simulink model "sim_ismc"  (R2023b)
settings: Solver=ode1  StartTime=0.0  StopTime=2  FixedStep=0.0001  RelTol=1e-3
values from neighbouring files (symbols this model uses):
  dn_lim = -up_lim    (= -10)    [ai_smc.m]    (also in ismc.m; st_smc.m)
  k_smc_e = 1    [ismc.m]
  k_smc_ie = -5    [ismc.m]
  M = -2    [fsmc.m]    (also in ismc.m = 10)
  Te = 0.001    [ai_smc.m]    (also in fsmc.m; ismc.m; st_smc.m)
  Tm = 0.2    [ai_smc.m]    (also in fsmc.m; ismc.m; st_smc.m)
  up_lim = 10    [ai_smc.m]    (also in ismc.m; st_smc.m)
settings Model: Creator=HP  LastModifiedBy=HP

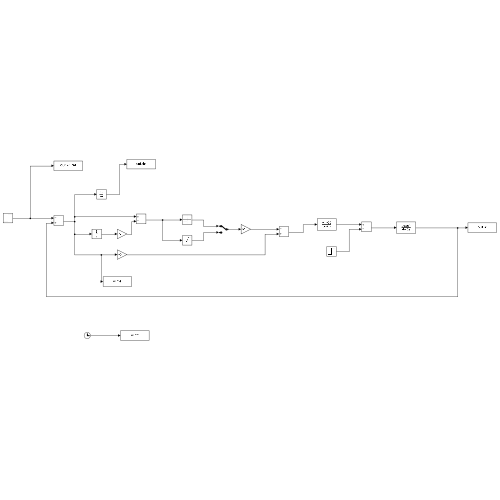
[thumbnail: Simulink's stored preview of the top-level diagram]
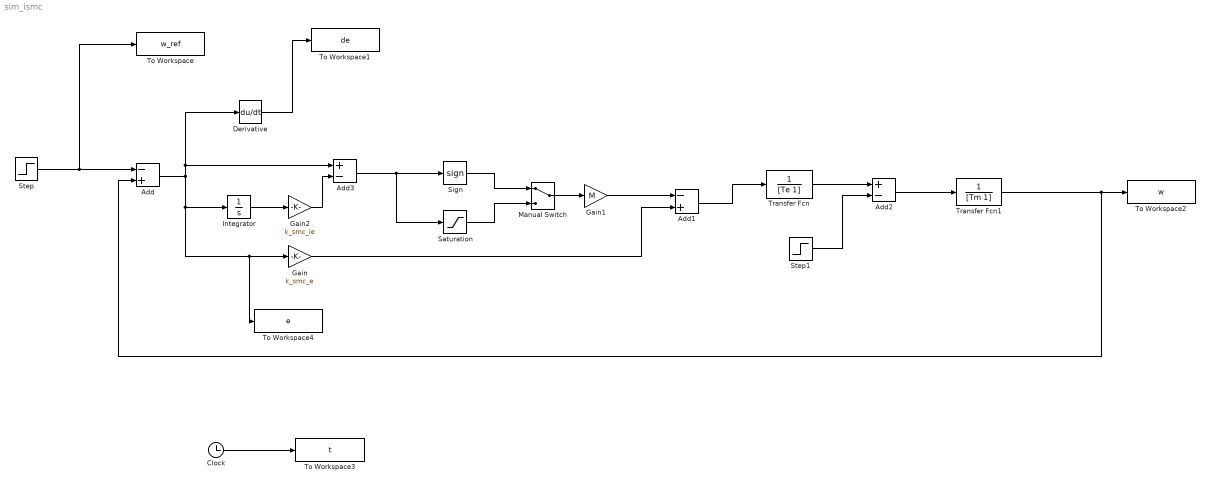
== system sim_ismc ==
  Add : Sum  Inputs=-+
  Add1 : Sum  Inputs=-+
  Add2 : Sum  Inputs=+-
  Add3 : Sum  Inputs=+-
  Clock : Clock
  Derivative : Derivative
  Gain : Gain  Gain=k_smc_e
  Gain1 : Gain  Gain=M
  Gain2 : Gain  Gain=k_smc_ie
  Integrator : Integrator
  Manual Switch : ManualSwitch
  Saturation : Saturate  UpperLimit=up_lim  LowerLimit=dn_lim
  Sign : Signum
  Step : Step  Time=0.1  SampleTime=0
  Step1 : Step  SampleTime=0
  To Workspace : ToWorkspace  VariableName=w_ref  SaveFormat=Timeseries  SampleTime=-1
  To Workspace1 : ToWorkspace  VariableName=de  SaveFormat=Timeseries  SampleTime=-1
  To Workspace2 : ToWorkspace  VariableName=w  SaveFormat=Timeseries  SampleTime=-1
  To Workspace3 : ToWorkspace  VariableName=t  SaveFormat=Timeseries  SampleTime=-1
  To Workspace4 : ToWorkspace  VariableName=e  SaveFormat=Timeseries  SampleTime=-1
  Transfer Fcn : TransferFcn  Denominator=[Te 1]
  Transfer Fcn1 : TransferFcn  Denominator=[Tm 1]
  wires:
  Step/1 -> Add/1, To Workspace/1
  Add/1 -> Derivative/1, Add3/1, Integrator/1, To Workspace4/1, Gain/1
  Derivative/1 -> To Workspace1/1
  Transfer Fcn/1 -> Add2/1
  Add2/1 -> Transfer Fcn1/1
  Transfer Fcn1/1 -> Add/2, To Workspace2/1
  Clock/1 -> To Workspace3/1
  Step1/1 -> Add2/2
  Saturation/1 -> Manual Switch/2
  Sign/1 -> Manual Switch/1
  Manual Switch/1 -> Gain1/1
  Integrator/1 -> Gain2/1
  Gain2/1 -> Add3/2
  Add3/1 -> Sign/1, Saturation/1
  Gain1/1 -> Add1/1
  Gain/1 -> Add1/2
  Add1/1 -> Transfer Fcn/1
